simulink model "demodulation_c"  (R2021a)
settings: Solver=FixedStepAuto  StartTime=0.0  StopTime=0.1  RelTol=1e-3
libraries: dspsrcs4 x5, dsparch4 x1
settings Model: Creator=jimmypan  LastModifiedBy=jimmypan

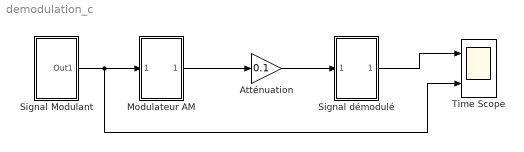
== system demodulation_c ==
  "Atténuation " : Gain  Gain=0.1
  Modulateur AM : Subsystem
  Signal Modulant : Subsystem
  "Signal démodulé " : Subsystem
  Time Scope : Scope  NumInputPorts=2
  wires:
  Modulateur AM/1(Out1) -> "Atténuation "/1
  Signal Modulant/1(Out1) -> Time Scope/2, Modulateur AM/1(In1)
  "Atténuation "/1 -> "Signal démodulé "/1(In1)
  "Signal démodulé "/1(Out1) -> Time Scope/1

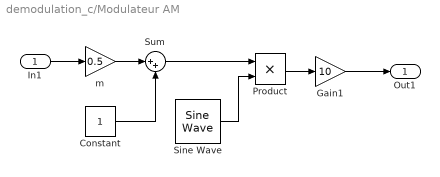
== system demodulation_c/Modulateur AM ==
  In1 : Inport
  Constant : Constant
  Gain1 : Gain  Gain=10
  Product : Product
  Sine Wave : dspsrcs4/Sine Wave  Amplitude=1  Frequency=20000  Phase=pi/2  SampleMode=Discrete  OutComplex=Real  CompMethod=Trigonometric fcn  TableSize=Speed  SampleTime=1/1000000  SamplesPerFrame=1  ResetState=Restart at time zero  OutputFrames=off  dataType=double  wordLen=16  udDataType=sfix(16)  fracBitsMode=Best precision  numFracBits=15  OutDataTypeStr=double  LastOutDataTypeStr=double
  Sum : Sum  Inputs=|++
  m : Gain  Gain=0.5
  Out1 : Outport
  wires:
  Sine Wave/1 -> Product/2
  Product/1 -> Gain1/1
  Gain1/1 -> Out1/1
  Sum/1 -> Product/1
  Constant/1 -> Sum/2
  In1/1 -> m/1
  m/1 -> Sum/1

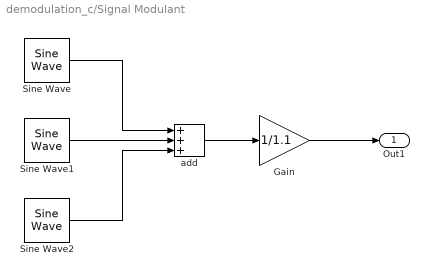
== system demodulation_c/Signal Modulant ==
  Gain : Gain  Gain=1/1.1
  Sine Wave : dspsrcs4/Sine Wave  Amplitude=1  Frequency=500  Phase=0  SampleMode=Discrete  OutComplex=Real  CompMethod=Trigonometric fcn  TableSize=Speed  SampleTime=1/1000000  SamplesPerFrame=1  ResetState=Restart at time zero  OutputFrames=off  dataType=double  wordLen=16  udDataType=sfix(16)  fracBitsMode=Best precision  numFracBits=15  OutDataTypeStr=double  LastOutDataTypeStr=double
  Sine Wave1 : dspsrcs4/Sine Wave  Amplitude=0.5  Frequency=1500  Phase=0  SampleMode=Discrete  OutComplex=Real  CompMethod=Trigonometric fcn  TableSize=Speed  SampleTime=1/1000000  SamplesPerFrame=1  ResetState=Restart at time zero  OutputFrames=off  dataType=double  wordLen=16  udDataType=sfix(16)  fracBitsMode=Best precision  numFracBits=15  OutDataTypeStr=double  LastOutDataTypeStr=double
  Sine Wave2 : dspsrcs4/Sine Wave  Amplitude=0.2  Frequency=2500  Phase=0  SampleMode=Discrete  OutComplex=Real  CompMethod=Trigonometric fcn  TableSize=Speed  SampleTime=1/1000000  SamplesPerFrame=1  ResetState=Restart at time zero  OutputFrames=off  dataType=double  wordLen=16  udDataType=sfix(16)  fracBitsMode=Best precision  numFracBits=15  OutDataTypeStr=double  LastOutDataTypeStr=double
  add : Sum  Inputs=+++
  Out1 : Outport
  wires:
  add/1 -> Gain/1
  Sine Wave2/1 -> add/3
  Sine Wave/1 -> add/1
  Sine Wave1/1 -> add/2
  Gain/1 -> Out1/1

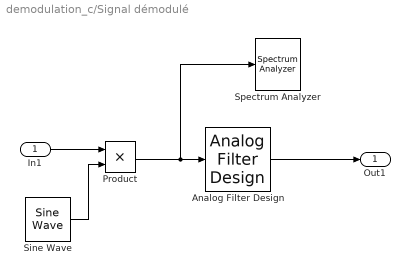
== system demodulation_c/Signal démodulé  ==
  In1 : Inport
  Analog Filter Design : dsparch4/Analog Filter Design  method=Butterworth  filttype=Lowpass  N=8  Wlo=130000  Whi=80  Rp=2  Rs=40
  Product : Product
  Sine Wave : dspsrcs4/Sine Wave  Amplitude=1  Frequency=20000  Phase=pi/2  SampleMode=Discrete  OutComplex=Real  CompMethod=Trigonometric fcn  TableSize=Speed  SampleTime=1/1000000  SamplesPerFrame=1  ResetState=Restart at time zero  OutputFrames=off  dataType=double  wordLen=16  udDataType=sfix(16)  fracBitsMode=Best precision  numFracBits=15  OutDataTypeStr=double  LastOutDataTypeStr=double
  Spectrum Analyzer : SpectrumAnalyzer
  Out1 : Outport
  wires:
  Sine Wave/1 -> Product/2
  In1/1 -> Product/1
  Analog Filter Design/1 -> Out1/1
  Product/1 -> Spectrum Analyzer/1, Analog Filter Design/1
